simulink model "model_nonlinear"  (R2024a)
settings: Solver=ode4  StartTime=0  StopTime=1.1  FixedStep=0.01  RelTol=1e-3
undefined symbols (not defined in the file or in its folder): A, B, b10, b20, f0, g0, gamma0, m0, r_max, r_min, theta_max, theta_min, x10, x20, x30, x40
settings Model: Creator=brzan  LastModifiedBy=brzan

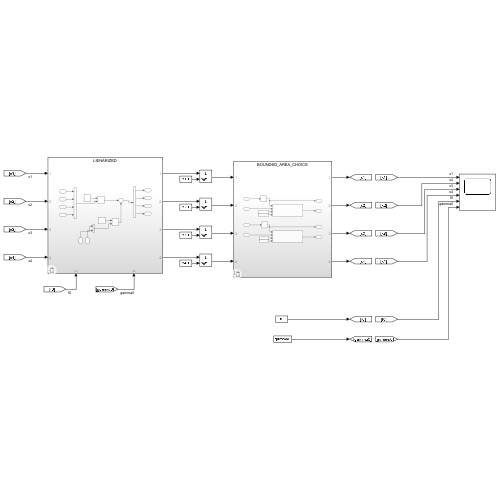
[thumbnail: Simulink's stored preview of the top-level diagram]
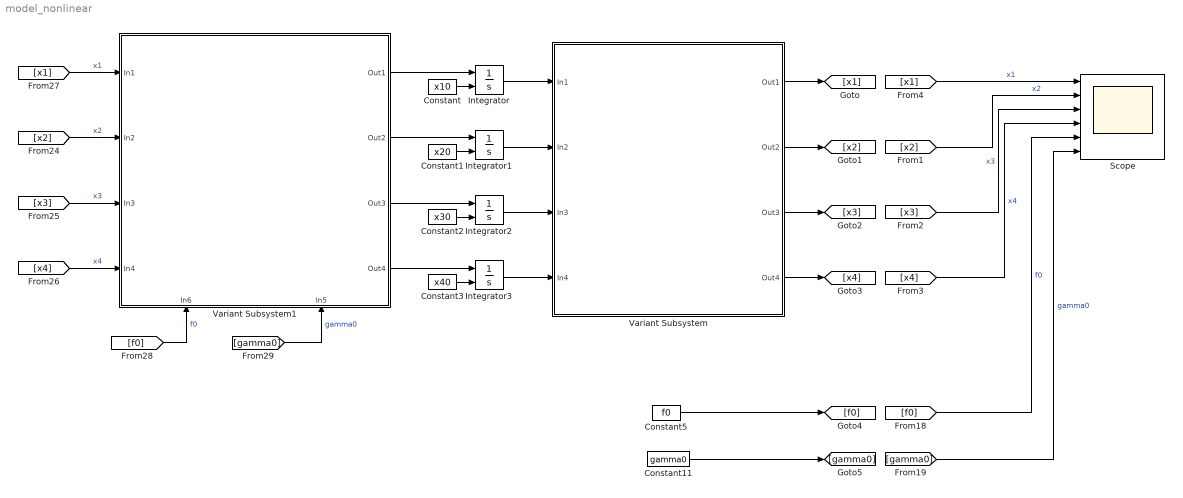
== system model_nonlinear ==
  Constant : Constant  Value=x10
  Constant1 : Constant  Value=x20
  Constant11 : Constant  Value=gamma0
  Constant2 : Constant  Value=x30
  Constant3 : Constant  Value=x40
  Constant5 : Constant  Value=f0
  Integrator{,1..3} (4 alike) : Integrator  InitialConditionSource=external
  Scope : Scope  NumInputPorts=6
  Variant Subsystem : Subsystem  Variant=on
  Variant Subsystem1 : Subsystem  Variant=on
      settings: PortSchema="{\"entries\":[{\"content\":{\"sides\":[{\"content\":{\"connectorIds\":[\"In1\",\"In2\",\"In3\",\"In4\"]},\"type\":\"ConnectorPlacement.EquallySpacedRectSide\",\"uuid\":\"20baa648-9fec-40ba-a5dd-b726b5049ca9\"},{\"content\":{\"connectorIds\":[\"Out1\",\"Out2\",\"Out3\",\"Out4\"],\"side\":\"RIGHT\"},\"type\":\"ConnectorPlacement.EquallySpacedRectSide\",\"uuid\":\"d1708c40-bdf1-40a1-9dcb-6b5286585c6c\"},{\"content\":{\"side\":\"TOP\"},\"type\":\"ConnectorPlacement.EquallySpacedRectSide\",\"uuid\":\"aebd4e89-1553-4225-9d19-2f71b97a4ddc\"},{\"content\":{\"connectorIds\":[\"In5\",\"In6\"],\"side\":\"BOTTOM\"},\"type\":\"ConnectorPlacement.EquallySpacedRectSide\",\"uuid\":\"b4da0231-142f-45ef-b4b6-14a0c0aeda15\"}]},\"type\":\"ConnectorPlacement.EquallySpacedConnector\",\"uuid\":\"cca832aa-4783-41c2-98ca-4452d2aff1fa\"}],\"packageUris\":[\"http://schema.mathworks.com/mf0/Connector/R2020b\"],\"version\":\"1.0\"}"
  wires:
  Constant/1 -> Integrator/2
  Constant1/1 -> Integrator1/2
  Constant2/1 -> Integrator2/2
  Constant3/1 -> Integrator3/2
  [x4] -> Scope/4  "x4"
  [x3] -> Scope/3  "x3"
  [x2] -> Scope/2  "x2"
  [x1] -> Scope/1  "x1"
  Constant5/1 -> [f0]
  Constant11/1 -> [gamma0]
  [f0] -> Scope/5  "f0"
  [gamma0] -> Scope/6  "gamma0"
  Integrator/1 -> Variant Subsystem/1(In1)
  Integrator1/1 -> Variant Subsystem/2(In2)
  Integrator2/1 -> Variant Subsystem/3(In3)
  Integrator3/1 -> Variant Subsystem/4(In4)
  Variant Subsystem/1(Out1) -> [x1]
  Variant Subsystem/2(Out2) -> [x2]
  Variant Subsystem/3(Out3) -> [x3]
  Variant Subsystem/4(Out4) -> [x4]
  Variant Subsystem1/1(Out1) -> Integrator/1
  Variant Subsystem1/2(Out2) -> Integrator1/1
  Variant Subsystem1/3(Out3) -> Integrator2/1
  Variant Subsystem1/4(Out4) -> Integrator3/1
  [x4] -> Variant Subsystem1/4(In4)  "x4"
  [x3] -> Variant Subsystem1/3(In3)  "x3"
  [x2] -> Variant Subsystem1/2(In2)  "x2"
  [x1] -> Variant Subsystem1/1(In1)  "x1"
  [f0] -> Variant Subsystem1/5(In6)  "f0"
  [gamma0] -> Variant Subsystem1/6(In5)  "gamma0"

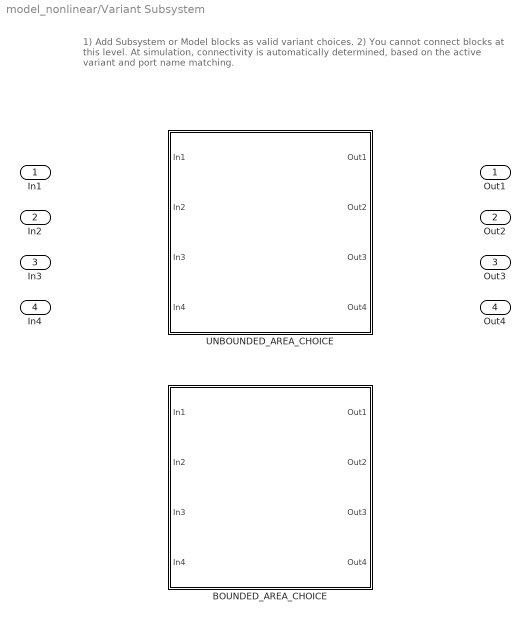
== system model_nonlinear/Variant Subsystem ==
  note: 1) Add Subsystem or Model blocks as valid variant choices.
      | 2) You cannot connect blocks at this level. At simulation, connectivity is automatically
      | determined, based on the active variant and port name matching.
  In1 : Inport
  In2 : Inport  Port=2
  In3 : Inport  Port=3
  In4 : Inport  Port=4
  BOUNDED_AREA_CHOICE : Subsystem  VariantControl="BOUNDARY_CHOICE == \"BOUNDED\""
  UNBOUNDED_AREA_CHOICE : Subsystem  VariantControl="BOUNDARY_CHOICE == \"UNBOUNDED\""
  Out1 : Outport
  Out2 : Outport  Port=2
  Out3 : Outport  Port=3
  Out4 : Outport  Port=4

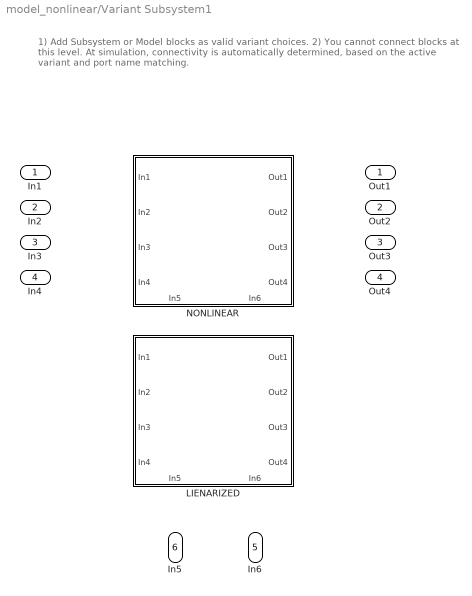
== system model_nonlinear/Variant Subsystem1 ==
  note: 1) Add Subsystem or Model blocks as valid variant choices.
      | 2) You cannot connect blocks at this level. At simulation, connectivity is automatically
      | determined, based on the active variant and port name matching.
  In1 : Inport
  In2 : Inport  Port=2
  In3 : Inport  Port=3
  In4 : Inport  Port=4
  In6 : Inport  Port=5
  In5 : Inport  Port=6
  LIENARIZED : Subsystem  VariantControl="MODEL_CHOICE == \"LINEARIZED\""
      settings: PortSchema="{\"entries\":[{\"content\":{\"sides\":[{\"content\":{\"connectorIds\":[\"In1\",\"In2\",\"In3\",\"In4\"]},\"type\":\"ConnectorPlacement.EquallySpacedRectSide\",\"uuid\":\"20baa648-9fec-40ba-a5dd-b726b5049ca9\"},{\"content\":{\"connectorIds\":[\"Out1\",\"Out2\",\"Out3\",\"Out4\"],\"side\":\"RIGHT\"},\"type\":\"ConnectorPlacement.EquallySpacedRectSide\",\"uuid\":\"d1708c40-bdf1-40a1-9dcb-6b5286585c6c\"},{\"content\":{\"side\":\"TOP\"},\"type\":\"ConnectorPlacement.EquallySpacedRectSide\",\"uuid\":\"aebd4e89-1553-4225-9d19-2f71b97a4ddc\"},{\"content\":{\"connectorIds\":[\"In5\",\"In6\"],\"side\":\"BOTTOM\"},\"type\":\"ConnectorPlacement.EquallySpacedRectSide\",\"uuid\":\"37909ba8-29a7-4181-9692-db8a229235b4\"}]},\"type\":\"ConnectorPlacement.EquallySpacedConnector\",\"uuid\":\"cca832aa-4783-41c2-98ca-4452d2aff1fa\"}],\"packageUris\":[\"http://schema.mathworks.com/mf0/Connector/R2020b\"],\"version\":\"1.0\"}"
  NONLINEAR : Subsystem  VariantControl="MODEL_CHOICE == \"NONLINEAR\""
      settings: PortSchema="{\"entries\":[{\"content\":{\"sides\":[{\"content\":{\"connectorIds\":[\"In1\",\"In2\",\"In3\",\"In4\"]},\"type\":\"ConnectorPlacement.EquallySpacedRectSide\",\"uuid\":\"20baa648-9fec-40ba-a5dd-b726b5049ca9\"},{\"content\":{\"connectorIds\":[\"Out1\",\"Out2\",\"Out3\",\"Out4\"],\"side\":\"RIGHT\"},\"type\":\"ConnectorPlacement.EquallySpacedRectSide\",\"uuid\":\"d1708c40-bdf1-40a1-9dcb-6b5286585c6c\"},{\"content\":{\"side\":\"TOP\"},\"type\":\"ConnectorPlacement.EquallySpacedRectSide\",\"uuid\":\"aebd4e89-1553-4225-9d19-2f71b97a4ddc\"},{\"content\":{\"connectorIds\":[\"In5\",\"In6\"],\"side\":\"BOTTOM\"},\"type\":\"ConnectorPlacement.EquallySpacedRectSide\",\"uuid\":\"37909ba8-29a7-4181-9692-db8a229235b4\"}]},\"type\":\"ConnectorPlacement.EquallySpacedConnector\",\"uuid\":\"cca832aa-4783-41c2-98ca-4452d2aff1fa\"}],\"packageUris\":[\"http://schema.mathworks.com/mf0/Connector/R2020b\"],\"version\":\"1.0\"}"
  Out1 : Outport
  Out2 : Outport  Port=2
  Out3 : Outport  Port=3
  Out4 : Outport  Port=4

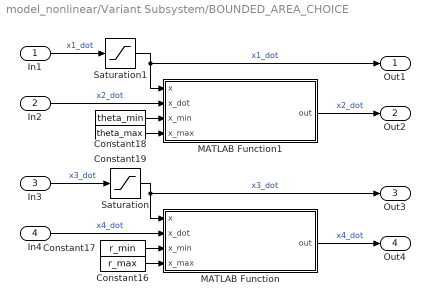
== system model_nonlinear/Variant Subsystem/BOUNDED_AREA_CHOICE ==
  In1 : Inport
  In2 : Inport  Port=2
  In3 : Inport  Port=3
  In4 : Inport  Port=4
  Constant16 : Constant  Value=r_max
  Constant17 : Constant  Value=r_min
  Constant18 : Constant  Value=theta_min
  Constant19 : Constant  Value=theta_max
  MATLAB Function : MATLAB Function  TreatAsAtomicUnit=on
  MATLAB Function1 : MATLAB Function  TreatAsAtomicUnit=on
  Saturation : Saturate  UpperLimit=r_max  LowerLimit=r_min
  Saturation1 : Saturate  UpperLimit=theta_max  LowerLimit=theta_min
  Out1 : Outport
  Out2 : Outport  Port=2
  Out3 : Outport  Port=3
  Out4 : Outport  Port=4
  wires:
  In3/1 -> Saturation/1  "x3_dot"
  Constant18/1 -> MATLAB Function1/3(x_min)
  In1/1 -> Saturation1/1  "x1_dot"
  Saturation1/1 -> Out1/1, MATLAB Function1/1(x)  "x1_dot"
  Saturation/1 -> Out3/1, MATLAB Function/1(x)  "x3_dot"
  Constant17/1 -> MATLAB Function/3(x_min)
  Constant16/1 -> MATLAB Function/4(x_max)
  Constant19/1 -> MATLAB Function1/4(x_max)
  MATLAB Function1/1(out) -> Out2/1  "x2_dot"
  In2/1 -> MATLAB Function1/2(x_dot)  "x2_dot"
  In4/1 -> MATLAB Function/2(x_dot)  "x4_dot"
  MATLAB Function/1(out) -> Out4/1  "x4_dot"

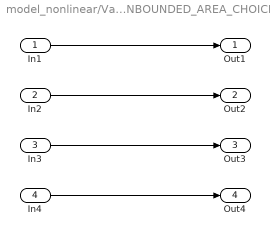
== system model_nonlinear/Variant Subsystem/UNBOUNDED_AREA_CHOICE ==
  In1 : Inport
  In2 : Inport  Port=2
  In3 : Inport  Port=3
  In4 : Inport  Port=4
  Out1 : Outport
  Out2 : Outport  Port=2
  Out3 : Outport  Port=3
  Out4 : Outport  Port=4
  wires:
  In1/1 -> Out1/1
  In2/1 -> Out2/1
  In3/1 -> Out3/1
  In4/1 -> Out4/1

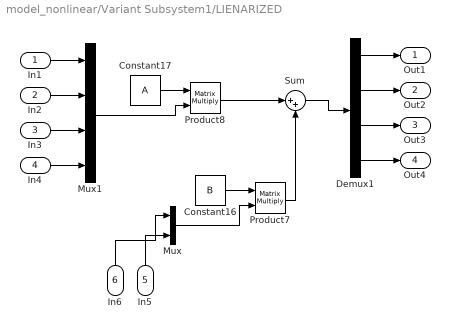
== system model_nonlinear/Variant Subsystem1/LIENARIZED ==
  In1 : Inport
  In2 : Inport  Port=2
  In3 : Inport  Port=3
  In4 : Inport  Port=4
  In5 : Inport  Port=5
  In6 : Inport  Port=6
  Constant16 : Constant  Value=B  VectorParams1D=off
  Constant17 : Constant  Value=A  VectorParams1D=off
  Demux1 : Demux
  Mux : Mux  Inputs=2
  Mux1 : Mux
  Product7 : Product  Multiplication=Matrix(*)
  Product8 : Product  Multiplication=Matrix(*)
  Sum : Sum  Inputs=|++
  Out1 : Outport
  Out2 : Outport  Port=2
  Out3 : Outport  Port=3
  Out4 : Outport  Port=4
  wires:
  Mux1/1 -> Product8/2
  Sum/1 -> Demux1/1
  Product8/1 -> Sum/1
  Constant17/1 -> Product8/1
  Product7/1 -> Sum/2
  Constant16/1 -> Product7/1
  Mux/1 -> Product7/2
  In4/1 -> Mux1/4
  In3/1 -> Mux1/3
  In2/1 -> Mux1/2
  In1/1 -> Mux1/1
  In6/1 -> Mux/1
  In5/1 -> Mux/2
  Demux1/1 -> Out1/1
  Demux1/2 -> Out2/1
  Demux1/3 -> Out3/1
  Demux1/4 -> Out4/1

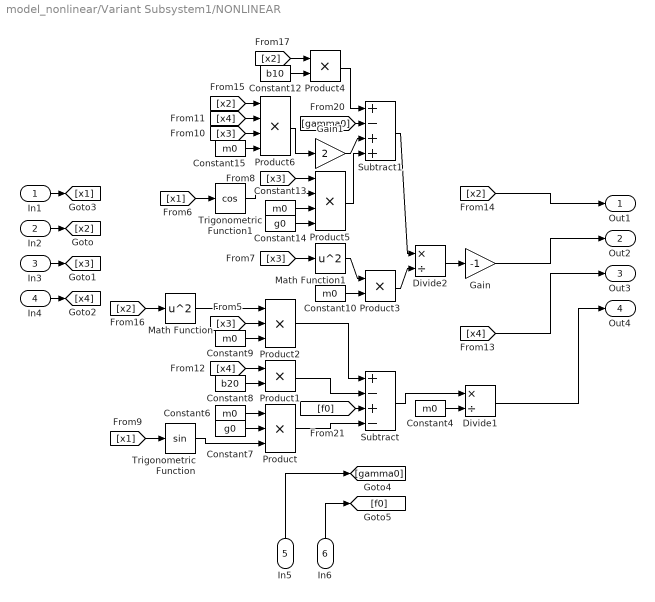
== system model_nonlinear/Variant Subsystem1/NONLINEAR ==
  In1 : Inport
  In2 : Inport  Port=2
  In3 : Inport  Port=3
  In4 : Inport  Port=4
  In5 : Inport  Port=5
  In6 : Inport  Port=6
  Constant{4,6,9..10,13,15} (6 alike) : Constant  Value=m0
  Constant12 : Constant  Value=b10
  Constant14 : Constant  Value=g0
  Constant7 : Constant  Value=g0
  Constant8 : Constant  Value=b20
  Divide1 : Product  Inputs=*/
  Divide2 : Product  Inputs=*/
  Gain : Gain  Gain=-1
  Gain1 : Gain  Gain=2
  Math Function : Math  Operator=square
  Math Function1 : Math  Operator=square
  Product : Product  Inputs=3
  Product1 : Product
  Product2 : Product  Inputs=3
  Product3 : Product
  Product4 : Product
  Product5 : Product  Inputs=4
  Product6 : Product  Inputs=4
  Subtract : Sum  Inputs=+-+-
  Subtract1 : Sum  Inputs=+-++
  Trigonometric Function : Trigonometry
  Trigonometric Function1 : Trigonometry  Operator=cos
  Out1 : Outport
  Out2 : Outport  Port=2
  Out3 : Outport  Port=3
  Out4 : Outport  Port=4
  wires:
  Constant7/1 -> Product/2
  Product/1 -> Subtract/4
  Subtract1/1 -> Divide2/1
  Product2/1 -> Subtract/1
  Constant15/1 -> Product6/4
  [f0] -> Subtract/3
  [x2] -> Out1/1
  Constant9/1 -> Product2/3
  [x3] -> Product2/2
  [gamma0] -> Subtract1/2
  Constant12/1 -> Product4/2
  Product1/1 -> Subtract/2
  Math Function1/1 -> Product3/1
  Constant10/1 -> Product3/2
  Divide2/1 -> Gain/1
  Subtract/1 -> Divide1/1
  Product3/1 -> Divide2/2
  Gain1/1 -> Subtract1/3
  [x2] -> Product4/1
  Constant6/1 -> Product/1
  Constant13/1 -> Product5/3
  [x1] -> Trigonometric Function/1
  Product5/1 -> Subtract1/4
  Product4/1 -> Subtract1/1
  Math Function/1 -> Product2/1
  [x4] -> Product6/2
  Gain/1 -> Out2/1
  Constant4/1 -> Divide1/2
  Trigonometric Function/1 -> Product/3
  [x4] -> Product1/1
  Product6/1 -> Gain1/1
  [x2] -> Math Function/1
  [x3] -> Product5/1
  Constant8/1 -> Product1/2
  [x2] -> Product6/1
  Trigonometric Function1/1 -> Product5/2
  [x1] -> Trigonometric Function1/1
  [x3] -> Math Function1/1
  Constant14/1 -> Product5/4
  [x4] -> Out3/1
  Divide1/1 -> Out4/1
  [x3] -> Product6/3
  In2/1 -> [x2]
  In3/1 -> [x3]
  In4/1 -> [x4]
  In1/1 -> [x1]
  In6/1 -> [f0]
  In5/1 -> [gamma0]

== matlab function model_nonlinear/Variant Subsystem/BOUNDED_AREA_CHOICE/MATLAB Function1 ==
  data: x input; out output; x_dot input; x_min input; x_max input
function out = saturate_velocity(x, x_dot, x_min, x_max)
    if (x >= x_max && x_dot > 0) || (x <= x_min && x_dot < 0)
        out = 0;
    else
        out = x_dot;
    end
end

== matlab function model_nonlinear/Variant Subsystem/BOUNDED_AREA_CHOICE/MATLAB Function ==
  data: x input; out output; x_dot input; x_min input; x_max input
function out = saturate_velocity(x, x_dot, x_min, x_max)
    if (x >= x_max && x_dot > 0) || (x <= x_min && x_dot < 0)
        out = 0;
    else
        out = x_dot;
    end
end
